simulink model "Kinematics"  (R2024b)
settings: Solver=VariableStepAuto  StartTime=0.0  StopTime=10.0  RelTol=1e-3
undefined symbols (not defined in the file): robotGoal, startPose
libraries: robotmobilelib x1
settings Model: DataDictionary=DataDictionary.sldd  Creator=charber  LastModifiedBy=tsamak
settings ModelReferenceCC: ModelReferenceMinAlgLoopOccurrences=on

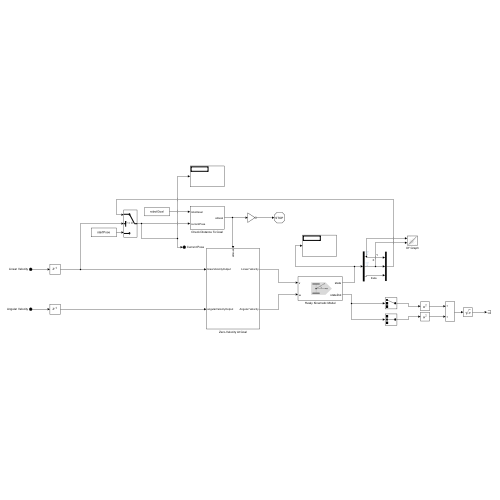
[thumbnail: Simulink's stored preview of the top-level diagram]
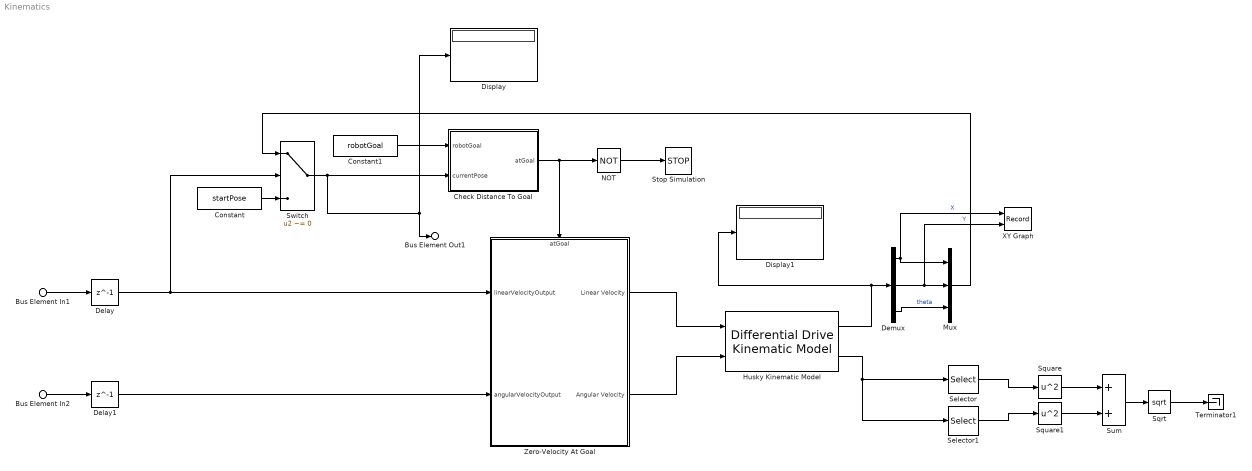
== system Kinematics ==
  Bus Element In1 : Inport  PortName=Linear Velocity
  Bus Element In2 : Inport  Port=2  PortName=Angular Velocity
  Check Distance To Goal : Subsystem
  Constant : Constant  Value=startPose
  Constant1 : Constant  Value=robotGoal
  Delay : Delay  DelayLength=1
  Delay1 : Delay  DelayLength=1
  Demux : Demux  Outputs=3
  Display : Display
  Display1 : Display
  Husky Kinematic Model : robotmobilelib/Differential Drive Kinematic Model  VehicleInputs=Vehicle Speed & Heading Angular Velocity  WheelRadius=0.27/2  WheelSpeedRange=[-inf inf]  TrackWidth=0.52  InitialState=[0; 0; 0]  SimulateUsing=Interpreted execution
  Mux : Mux  Inputs=3
  NOT : Logic  Operator=NOT  IconShape=distinctive  AllPortsSameDT=off  OutDataTypeStr=boolean
  Selector : Selector  InputPortWidth=3  IndexOptions=Index vector (dialog)  Indices=[1]  OutputSizes=1
  Selector1 : Selector  InputPortWidth=3  IndexOptions=Index vector (dialog)  Indices=[2]  OutputSizes=1
  Sqrt : Sqrt
  Square : Math  Operator=square
  Square1 : Math  Operator=square
  Stop Simulation : Stop
  Sum : Sum
  Switch : Switch  Criteria=u2 ~= 0  SaturateOnIntegerOverflow=off  InputSameDT=off
  Terminator1 : Terminator
  XY Graph : Record  FileSettingsInternal="{\"entries\":[{\"content\":{\"excelSettings\":{\"content\":{},\"type\":\"Streamout.ExcelSettings\"}},\"type\":\"Streamout.FileSettingStorage\",\"uuid\":\"\"}],\"packageUris\":[\"http:\\/\\/schema.mathworks.com\\/mf0\\/streamout_blocks\\/R2020a\"],\"version\":\"1.0\"}"  Layout=[1 1]  SignalsInternal="{\"entries\":[{\"content\":{},\"type\":\"RecordBlkView.InputSignals\",\"uuid\":\"\"}],\"packageUris\":[\"http:\\/\\/schema.mathworks.com\\/mf0\\/streamout_blocks\\/R2020a\"],\"version\":\"1.0\"}"  VisualizationBindings="{\"xyplotplugin\":{\"info\":[{\"series\":[],\"subplotID\":1}]}}"  CompatibilityTag=XY
  Zero-Velocity At Goal : Subsystem
      settings: PortSchema="{\"entries\":[{\"content\":{\"sides\":[{\"content\":{\"connectorIds\":[\"In1\",\"In2\"]},\"type\":\"ConnectorPlacement.EquallySpacedRectSide\",\"uuid\":\"d6ef090c-8691-4f8e-808e-16a05b1c931f\"},{\"content\":{\"connectorIds\":[\"Out1\",\"Out2\"],\"side\":\"RIGHT\"},\"type\":\"ConnectorPlacement.EquallySpacedRectSide\",\"uuid\":\"2ae6408e-e944-4e5d-bf23-2707e82d0ba7\"},{\"content\":{\"connectorIds\":[\"In3\"],\"side\":\"TOP\"},\"type\":\"ConnectorPlacement.EquallySpacedRectSide\",\"uuid\":\"29270005-91b8-4dcb-ad7c-17893aa9f4c0\"}]},\"type\":\"ConnectorPlacement.EquallySpacedConnector\",\"uuid\":\"a9fc078d-7ce2-488f-9666-d3d979ba1bbe\"}],\"packageUris\":[\"http://schema.mathworks.com/mf0/Connector/R2020b\"],\"version\":\"1.0\"}"
  Bus Element Out1 : Outport  PortName=Current Pose
  wires:
  Demux/3 -> Mux/3  "theta"
  Selector1/1 -> Square1/1
  Constant/1 -> Switch/3
  Constant1/1 -> Check Distance To Goal/1(robotGoal)
  Zero-Velocity At Goal/1(Linear Velocity) -> Husky Kinematic Model/1
  Square1/1 -> Sum/2
  Mux/1 -> Switch/1
  Bus Element In1/1 -> Delay/1
  NOT/1 -> Stop Simulation/1
  Check Distance To Goal/1(atGoal) -> Zero-Velocity At Goal/3(atGoal), NOT/1
  Selector/1 -> Square/1
  Demux/2 -> Mux/2, XY Graph/2  "Y"
  Square/1 -> Sum/1
  Husky Kinematic Model/1 -> Demux/1, Display1/1
  Demux/1 -> XY Graph/1, Mux/1  "X"
  Bus Element In2/1 -> Delay1/1
  Switch/1 -> Display/1, Bus Element Out1/1, Check Distance To Goal/2(currentPose)
  Sqrt/1 -> Terminator1/1
  Husky Kinematic Model/2 -> Selector1/1, Selector/1
  Sum/1 -> Sqrt/1
  Zero-Velocity At Goal/2(Angular Velocity) -> Husky Kinematic Model/2
  Delay/1 -> Switch/2, Zero-Velocity At Goal/1(linearVelocityOutput)
  Delay1/1 -> Zero-Velocity At Goal/2(angularVelocityOutput)

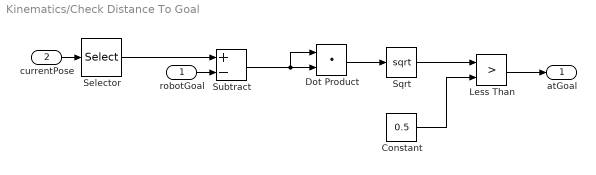
== system Kinematics/Check Distance To Goal ==
  robotGoal : Inport
  currentPose : Inport  Port=2
  Constant : Constant  Value=0.5
  Dot Product : DotProduct  OutDataTypeStr=Inherit: Inherit via internal rule
  Less Than : RelationalOperator  Operator=>  OutDataTypeStr=boolean  RndMeth=Simplest  InputSameDT=off
  Selector : Selector  InputPortWidth=3  IndexOptions=Index vector (dialog)  Indices=[1 2]  OutputSizes=1
  Sqrt : Sqrt
  Subtract : Sum  Inputs=+-
  atGoal : Outport
  wires:
  robotGoal/1 -> Subtract/2
  Dot Product/1 -> Sqrt/1
  Constant/1 -> Less Than/2
  currentPose/1 -> Selector/1
  Less Than/1 -> atGoal/1
  Sqrt/1 -> Less Than/1
  Subtract/1 -> Dot Product/1, Dot Product/2
  Selector/1 -> Subtract/1

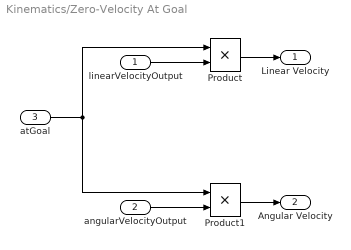
== system Kinematics/Zero-Velocity At Goal ==
  linearVelocityOutput : Inport
  angularVelocityOutput : Inport  Port=2
  atGoal : Inport  Port=3
  Product : Product
  Product1 : Product
  Linear Velocity : Outport  OutDataTypeStr=double
  Angular Velocity : Outport  Port=2  OutDataTypeStr=double
  wires:
  atGoal/1 -> Product1/1, Product/1
  angularVelocityOutput/1 -> Product1/2
  linearVelocityOutput/1 -> Product/2
  Product/1 -> Linear Velocity/1
  Product1/1 -> Angular Velocity/1
